simulink model "pcm_dieubien"  (R2023a)
settings: Solver=VariableStepAuto  StartTime=0.0  StopTime=1  RelTol=1e-3
libraries: simulink x1, dspsigops x1, dspquant2 x1
settings Model: Creator=dung  LastModifiedBy=dung

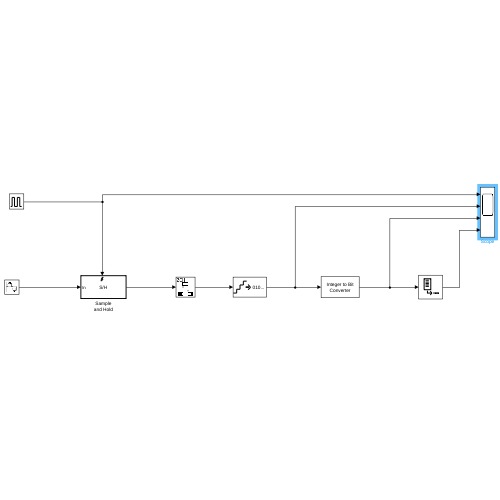
[thumbnail: Simulink's stored preview of the top-level diagram]
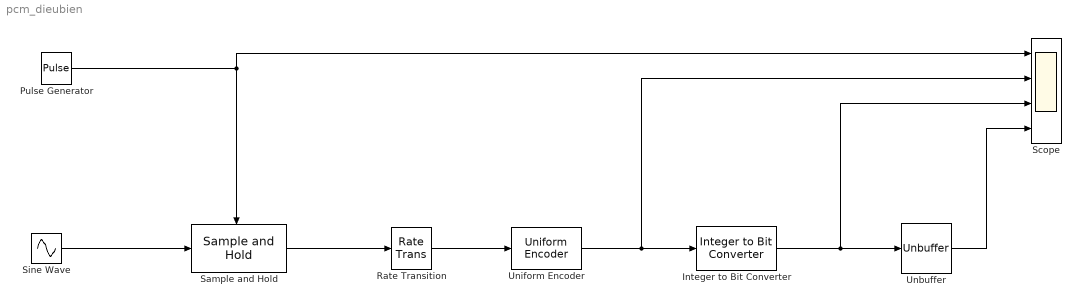
== system pcm_dieubien ==
  Integer to Bit Converter : simulink/Logic and Bit Operations/Integer to Bit Converter  nbits=8  signedInputValues=Unsigned  bitOrder=MSB first  outDtype=Inherit via internal rule
  Pulse Generator : DiscretePulseGenerator  PulseType=Time based  Period=1/8000  PulseWidth=50
  Rate Transition : RateTransition  OutPortSampleTime=1/8000
  Sample and Hold : dspsigops/Sample and Hold  trig=Rising edge  initCond=0  latchinput=off
  Scope : Scope  NumInputPorts=4
  Sine Wave : Sin  Frequency=2*pi*3000  SampleTime=1/64000
  Unbuffer : Unbuffer
  Uniform Encoder : dspquant2/Uniform Encoder  peak=1  bits=8  otype=Unsigned integer
  wires:
  Sample and Hold/1 -> Rate Transition/1
  Rate Transition/1 -> Uniform Encoder/1
  Uniform Encoder/1 -> Scope/2, Integer to Bit Converter/1
  Integer to Bit Converter/1 -> Scope/3, Unbuffer/1
  Unbuffer/1 -> Scope/4
  Pulse Generator/1 -> Sample and Hold/Trigger, Scope/1
  Sine Wave/1 -> Sample and Hold/1
